simulink model "Tobillo_Protesico_Control_v6"  (R2026a)
settings: Solver=ode45

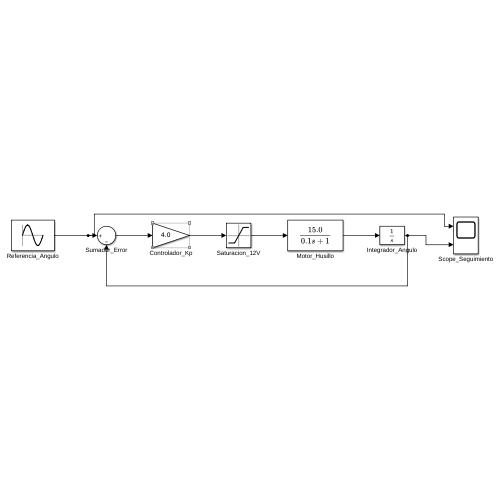
[thumbnail: Simulink's stored preview of the top-level diagram]
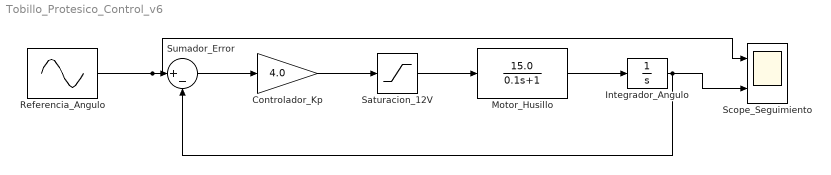
== system Tobillo_Protesico_Control_v6 ==
  Controlador_Kp : Gain  Gain=4.0
  Integrador_Angulo : Integrator  InitialCondition=0.0
  Motor_Husillo : TransferFcn  Numerator=[15.0]  Denominator=[0.1 1]
  Referencia_Angulo : Sin  Amplitude=10.0  Frequency=2*pi*0.5  SampleTime=0
  Saturacion_12V : Saturate  UpperLimit=12.0  LowerLimit=-12.0
  Scope_Seguimiento : Scope  NumInputPorts=2
      settings: ActiveDisplayYMinimum=-20.737582648331681  ActiveDisplayYMaximum=15.103214906230573
  Sumador_Error : Sum  Inputs=|+-
  wires:
  Referencia_Angulo/1 -> Scope_Seguimiento/1, Sumador_Error/1
  Sumador_Error/1 -> Controlador_Kp/1
  Controlador_Kp/1 -> Saturacion_12V/1
  Saturacion_12V/1 -> Motor_Husillo/1
  Motor_Husillo/1 -> Integrador_Angulo/1
  Integrador_Angulo/1 -> Scope_Seguimiento/2, Sumador_Error/2
